simulink model "Navigation_Simple"  (R2016b)
settings: Solver=VariableStepAuto  StartTime=0.0  StopTime=10.0  RelTol=1e-3
values from neighbouring files (symbols this model uses):
  Env =     [UAV_modelconfig.mat]
undefined symbols (not defined in the file or in its folder): TrimCondition
libraries: Navigation_Lib x3
settings Model: Creator=UAVLAB  LastModifiedBy=UAVLAB

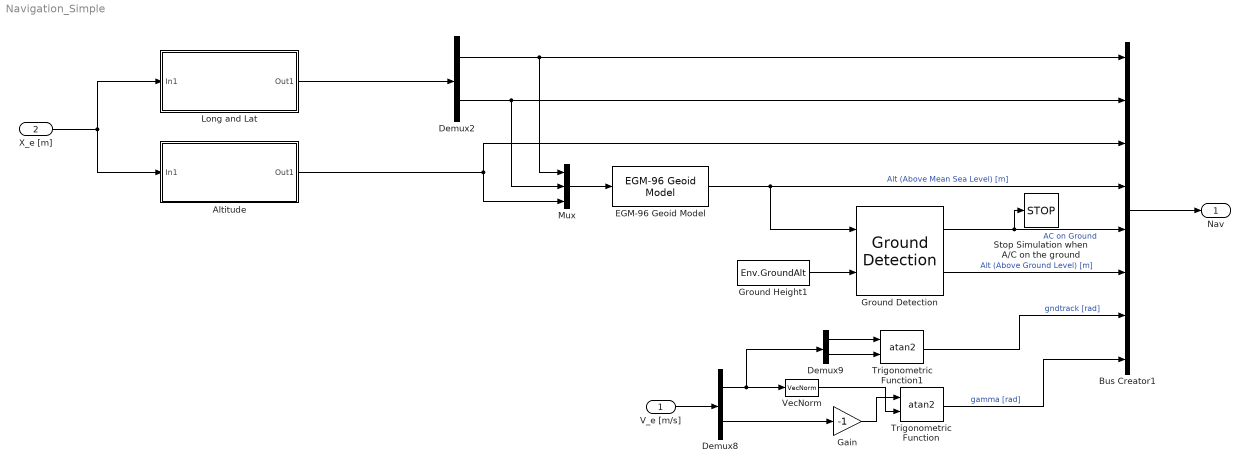
== system Navigation_Simple ==
  V_e [m/s] : Inport
  X_e [m] : Inport  Port=2
  Altitude : Subsystem
  Bus Creator1 : BusCreator  Inputs=8  OutDataTypeStr=Bus: Nav
      settings: InheritFromInputs=off
  Demux2 : Demux  Outputs=2
  Demux8 : Demux  Outputs=[2 1]
  Demux9 : Demux  Outputs=2
  EGM-96 Geoid Model : Navigation_Lib/Navigation/EGM-96 Geoid Model
  Gain : Gain  Gain=-1
  Ground Detection : Navigation_Lib/Navigation/Ground Detection
  Ground Height1 : Constant  Value=Env.GroundAlt
  Long and Lat : Subsystem
  Mux : Mux  Inputs=3
  Stop Simulation when A/C on the ground : Stop
  Trigonometric Function : Trigonometry  Operator=atan2
  Trigonometric Function1 : Trigonometry  Operator=atan2
  VecNorm : Navigation_Lib/Navigation/VecNorm
  Nav : Outport  OutDataTypeStr=Bus: Nav
  wires:
  Bus Creator1/1 -> Nav/1
  Demux2/1 -> Mux/1, Bus Creator1/1
  Demux2/2 -> Mux/2, Bus Creator1/2
  EGM-96 Geoid Model/1 -> Ground Detection/1, Bus Creator1/4  "Alt (Above Mean Sea Level) [m]"
  Ground Height1/1 -> Ground Detection/2
  Ground Detection/1 -> Stop Simulation when A/C on the ground/1, Bus Creator1/5  "AC on Ground"
  V_e [m/s]/1 -> Demux8/1
  Demux8/2 -> Gain/1
  VecNorm/1 -> Trigonometric Function/2
  Trigonometric Function/1 -> Bus Creator1/8  "gamma [rad]"
  Demux9/2 -> Trigonometric Function1/2
  Trigonometric Function1/1 -> Bus Creator1/7  "gndtrack [rad]"
  Demux8/1 -> VecNorm/1, Demux9/1
  Demux9/1 -> Trigonometric Function1/1
  Gain/1 -> Trigonometric Function/1
  Mux/1 -> EGM-96 Geoid Model/1
  Ground Detection/2 -> Bus Creator1/6  "Alt (Above Ground Level) [m]"
  X_e [m]/1 -> Altitude/1(In1), Long and Lat/1(In1)
  Altitude/1(Out1) -> Mux/3, Bus Creator1/3
  Long and Lat/1(Out1) -> Demux2/1

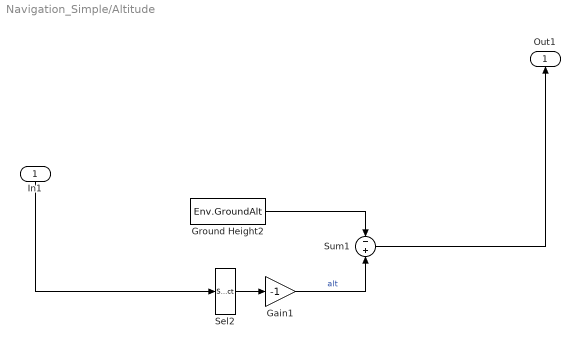
== system Navigation_Simple/Altitude ==
  In1 : Inport
  Gain1 : Gain  Gain=-1
  Ground Height2 : Constant  Value=Env.GroundAlt
  Sel2 : Selector  InputPortWidth=3  IndexOptions=Index vector (dialog)  Indices=3  OutputSizes=1
  Sum1 : Sum  Inputs=-+
  Out1 : Outport
  wires:
  In1/1 -> Sel2/1
  Gain1/1 -> Sum1/2  "alt"
  Sum1/1 -> Out1/1
  Sel2/1 -> Gain1/1
  Ground Height2/1 -> Sum1/1

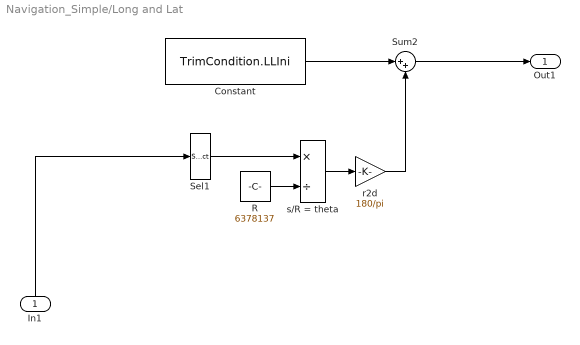
== system Navigation_Simple/Long and Lat ==
  In1 : Inport
  Constant : Constant  Value=TrimCondition.LLIni
  R : Constant  Value=6378137
  Sel1 : Selector  InputPortWidth=3  IndexOptions=Index vector (dialog)  Indices=[1 2]  OutputSizes=1
  Sum2 : Sum  Inputs=|++
  r2d : Gain  Gain=180/pi
  s/R = theta : Product  Inputs=*/
  Out1 : Outport
  wires:
  In1/1 -> Sel1/1
  R/1 -> s/R = theta/2
  Sel1/1 -> s/R = theta/1
  s/R = theta/1 -> r2d/1
  Sum2/1 -> Out1/1
  r2d/1 -> Sum2/2
  Constant/1 -> Sum2/1
